simulink model "das2_inv_for"  (Simulink 6.6)
settings: Solver=ode4  StartTime=0.0  StopTime=6  MaxStep=0.001  RelTol=1e-3
settings Model: Creator=chadwick  LastModifiedBy=admin  ExtModeAutoUpdateStatusClock=off  BufferReuse=off  ProdHWDeviceType=32-bit xPC Target (Intel Pentium)
settings DataIOCC: MaxDataPoints=20000  SaveFinalState=on  SaveOutput=off  SignalLogging=off  SaveTime=off
settings OptimizationCC: BlockReduction=off  InlineParams=on  OptimizeBlockIOStorage=off  BufferReuse=off  ExpressionFolding=off  LocalBlockOutputs=off
settings DebuggingCC: SignalResolutionControl=TryResolveAllWithWarning  MultiTaskDSMMsg=warning  MultiTaskCondExecSysMsg=none
settings HardwareCC: ProdIntDivRoundTo=Zero  ProdEndianess=LittleEndian  ProdHWDeviceType=32-bit xPC Target (Intel Pentium)
settings ModelReferenceCC: ModelReferenceNumInstancesAllowed=Single
settings RTWCC: SystemTargetFile=xpctarget.tlc  TemplateMakefile=xpc_default_tmf  Description=xPC Target  RetainRTWFile=on  ProcessScript=xpctarget_make_rtw_hook  CustomInclude=..\..\..\..\tools\sdbio\trunk\ ..\..\..\model\trunk\ ..\..\..\das1sim\trunk\  CustomSource=sdbio.c sdlib.c das1_d.c  IncludeERTFirstTime=on
settings xpcTargetCC: TargetFcnLib=ansi_tfl_tmw.mat  GenFloatMathFcnCalls=ANSI_C  PortableWordSizes=off  RL32LogBufSizeModifier=1000

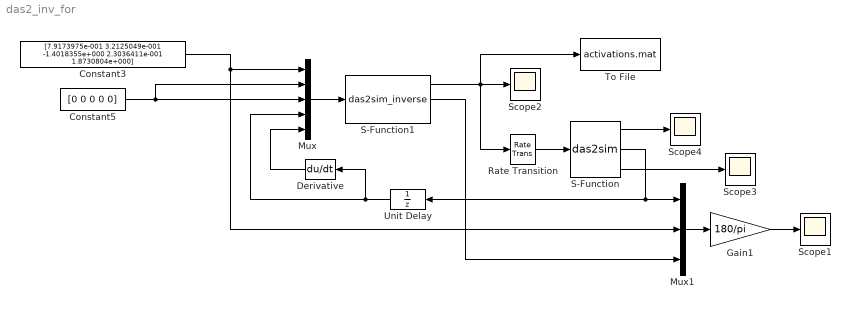
== system das2_inv_for ==
  Constant3 : Constant  Value="[7.9173975e-001  3.2125049e-001 -1.4018355e+000  2.3036411e-001  1.8730804e+000]"  SampleTime=0.001
  Constant5 : Constant  Value=[0 0 0 0 0]  SampleTime=0.001
  Derivative : Derivative  Orientation=left
  Gain1 : Gain  Gain=180/pi
  Mux : Mux  Inputs=5
  Mux1 : Mux  Inputs=3
  Rate Transition : RateTransition
  S-Function : S-Function  FunctionName=das2sim
  S-Function1 : S-Function  FunctionName=das2sim_inverse
  Scope{1..4} (4 alike) : Scope
      Scope1 settings: YMin=-100  YMax=125  SaveName=angles  DataFormat=Array
      Scope2 settings: YMin=0  YMax=1  SaveName=act  DataFormat=Array
      Scope3 settings: YMin=0  YMax=0.3
      Scope4 settings: YMin=-100  YMax=1500  SaveName=ScopeData3
  To File : ToFile  Filename=activations.mat  MatrixName=act
      settings: Decimation=10
  Unit Delay : UnitDelay  Orientation=left  X0="[7.9173975e-001  3.2125049e-001 -1.4018355e+000  2.3036411e-001  1.8730804e+000]"  SampleTime=-1
  wires:
  Gain1/1 -> Scope1/1
  Mux1/1 -> Gain1/1
  Derivative/1 -> Mux/5
  Unit Delay/1 -> Derivative/1, Mux/4
  S-Function1/1 -> Scope2/1, Rate Transition/1, To File/1
  S-Function1/2 -> Mux1/3
  S-Function/2 -> Mux1/1, Unit Delay/1
  S-Function/3 -> Scope3/1
  S-Function/1 -> Scope4/1
  Rate Transition/1 -> S-Function/1
  Constant5/1 -> Mux/2, Mux/3
  Constant3/1 -> Mux1/2, Mux/1
  Mux/1 -> S-Function1/1
